simulink model "trajectory_generation_ref_subsys_model_ref"  (R2022b)
settings: Solver=FixedStepAuto  StartTime=0.0  StopTime=10.0  FixedStep=param_global.Ta  RelTol=1e-3
settings Model: Creator=emu  LastModifiedBy=emu
settings OptimizationCC: ReuseModelBlockBuffer=on

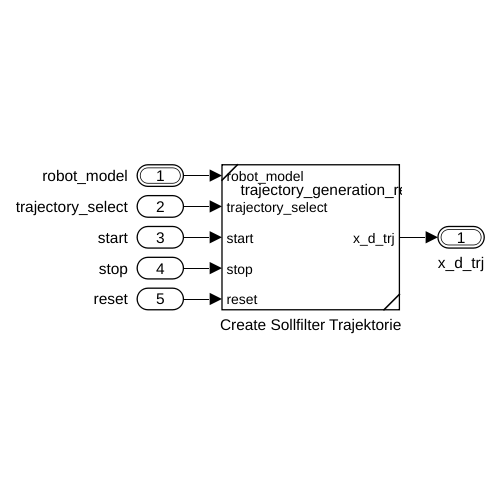
[thumbnail: Simulink's stored preview of the top-level diagram]
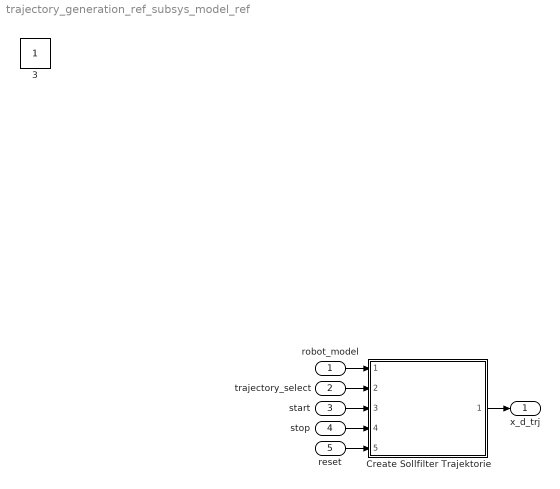
== system trajectory_generation_ref_subsys_model_ref ==
  robot_model : Inport  OutDataTypeStr=Bus: robot_model
  trajectory_select : Inport  Port=2
  start : Inport  Port=3
  stop : Inport  Port=4
  reset : Inport  Port=5
  Create Sollfilter Trajektorie : Subsystem  ReferencedSubsystem=trajectory_generation_ref_subsys
  x_d_trj : Outport  OutDataTypeStr=Bus: x_d
  3 : Constant  IOType=siggen
  wires:
  start/1 -> Create Sollfilter Trajektorie/3
  robot_model/1 -> Create Sollfilter Trajektorie/1
  stop/1 -> Create Sollfilter Trajektorie/4
  Create Sollfilter Trajektorie/1 -> x_d_trj/1
  reset/1 -> Create Sollfilter Trajektorie/5
  trajectory_select/1 -> Create Sollfilter Trajektorie/2
